simulink library "FlexBeamLib"  (R2019b)
settings: Solver=VariableStepAuto  StartTime=0.0  StopTime=10.0  RelTol=1e-3
undefined symbols (not defined in the file or in its folder): b, E, h, Izz, L, Mb, R, X, Y, Z
libraries: $bdroot x15, sm_lib x7
settings Model: Creator=tordaso  LastModifiedBy=tordaso

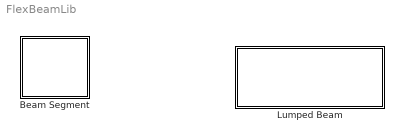
== system FlexBeamLib ==
  Beam Segment : Subsystem  mask{m=1, L=1, b=0.06, h=0.06, k=1000, c=10}
      mask prompts: m "Mass"; L "Length"; b "Width"; h "Height"; k "Joint Stiffness"; c "Joint Damping"
  Lumped Beam : Subsystem  mask{m=Mb(1), L=L(1), b=b(1), h=h(1), Izz=Izz(1), R=R, N=15, E=E}
      mask prompts: m "Mass"; L "Length"; b "Width"; h "Height"; R "Damping ratio"; N "Number of Elements"; E "E-Modulus"
      mask init:
      | % Get haandles of blocks and lines
      | blk = gcb;
      | blks = find_system(blk,...
      |     'LookUnderMasks','on',...
      |     'FollowLinks','on',...
      |     'FindAll', 'on'...
      | );
      | 
      | % Cleanup
      | for i = 2:length(blks)
      |     try
      |         type = get_param(blks(i), 'Type');
      |         name = get_param(blks(i), 'Name');
      |         
      |         if strcmp(type, 'line')
      |             delete_line(blks(i));
      |         end
      |         
      |         if strcmp(type, 'block')
      |             if strcmp(name, 'B')
      |                 hB = blks(i);
      |             elseif strcmp(name, 'F')
      |                 hF = blks(i);
      |             else
      |                 delete_block(blks(i));
      |             end
      |         end 
      |     end
      | end
      | 
      | % Beam segment paramters
      | mi = m/N;
      | Li = L/N;
      | bi = b;
      | hi = h;
      | ki = N*E*Izz/L;
      | ci = R*ki;
      | 
      | 
      | % Build N beam model
      | set_param([blk, '/B'], 'Position', flexlib.blockPos(0, 0, 30, 14));
      | for i = 1:N
      |     hBody = add_block('FlexBeamLib/Beam Segment',...
      |         [blk, '/body', num2str(i)],...
      |         'Position', flexlib.blockPos(70*i, 0, 40, 40)...
      |     );
      | 
      |     % Add lines
      |     if i > 1
      |         src = ['body', num2str(i-1), '/RConn1'];
      |         dst = ['body', num2str(i), '/LConn1'];
      |         
      |         add_line(blk, src, dst);
      |     end
      |     
      |     % Set parameters
      |     set_param(hBody, 'm', num2str(mi));
      |     set_param(hBody, 'L', num2str(Li));
      |     set_param(hBody, 'b', num2str(bi));
      |     set_param(hBody, 'h', num2str(hi));
      |     set_param(hBody, 'k', num2str(ki));
      |     set_param(hBody, 'c', num2str(ci));
      | 
      | end
      | 
      | % Move F
      | set_param([blk, '/F'], 'Position', flexlib.blockPos(70 + N*70, 0, 30, 14));
      | 
      | % Connect B and F
      | add_line(blk, 'B/RConn1', 'body1/LConn1');
      | add_line(blk, ['body', num2str(N), '/RConn1'], 'F/RConn1');

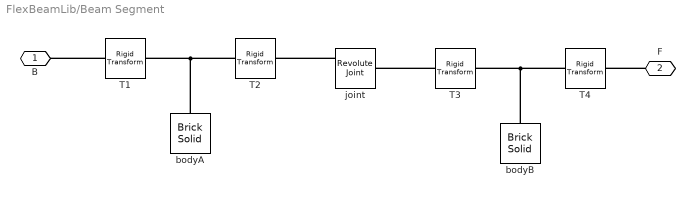
== system FlexBeamLib/Beam Segment ==
  T{1..4} (4 alike) : sm_lib/Frames and Transforms/Rigid Transform  TranslationMethod=Cartesian  TranslationStandardOffset=0  TranslationLengthUnit=m  TranslationStandardAxis=+Z  TranslationCartesianOffset=[L/4 0 0]  TranslationROffset=0  TranslationROffsetUnits=m  TranslationZOffset=0  TranslationZOffsetUnits=m  TranslationThetaOffset=0  TranslationThetaOffsetUnits=deg  RotationMethod=None  RotationAngleUnits=deg  RotationStandardAxis=+Z  RotationAngle=0.0  RotationArbitraryAxis=[0 0 1]  FollAlignAxisA=+X  BaseAlignAxisA=+Y  FollAlignAxisB=+Y  BaseAlignAxisB=+Z  RotationSequenceAxes=FollowerAxes  RotationSequence=XYX  RotationSequenceAngles=[0 0 0]  RotationSequenceAnglesUnits=deg  RotationMatrix=[1 0 0; 0 1 0; 0 0 1]
  bodyA : sm_lib/Body Elements/Brick Solid  GraphicAmbientColor=[0.15 0.15 0.15 1.0]  BasedOnType=Mass  BrickDimensions=[L/2 h b]  BrickDimensionUnits=m  CenterOfMass=[0 0 0]  CenterOfMassUnits=m  GraphicDiffuseColor=[0.0 0.0 0.0]  Density=1000  DensityUnits=kg/m^3  DoExposeReferenceFrame=on  GraphicEmissiveColor=[0.0 0.0 0.0 1.0]  ExportEntireGeometry=off  SerializedFrames=<Frames/>  MarkerShape=Sphere  MarkerSize=10  GraphicType=FromGeometry  InertiaType=CalculateFromGeometry  Mass=m  MassUnits=kg  MomentsOfInertia=[1 1 1]  MomentsOfInertiaUnits=kg*m^2  GraphicOpacity=1.0  ProductsOfInertia=[0 0 0]  ProductsOfInertiaUnits=kg*m^2  GraphicShininess=75  GraphicSpecularColor=[0.5 0.5 0.5 1.0]  GraphicVisPropType=SimpleVisualProperties
  bodyB : sm_lib/Body Elements/Brick Solid  GraphicAmbientColor=[0.15 0.15 0.15 1.0]  BasedOnType=Mass  BrickDimensions=[L/2 h b]  BrickDimensionUnits=m  CenterOfMass=[0 0 0]  CenterOfMassUnits=m  GraphicDiffuseColor=[1.0 1.0 0.0]  Density=1000  DensityUnits=kg/m^3  DoExposeReferenceFrame=on  GraphicEmissiveColor=[0.0 0.0 0.0 1.0]  ExportEntireGeometry=off  SerializedFrames=<Frames/>  MarkerShape=Sphere  MarkerSize=10  GraphicType=FromGeometry  InertiaType=CalculateFromGeometry  Mass=m  MassUnits=kg  MomentsOfInertia=[1 1 1]  MomentsOfInertiaUnits=kg*m^2  GraphicOpacity=1.0  ProductsOfInertia=[0 0 0]  ProductsOfInertiaUnits=kg*m^2  GraphicShininess=75  GraphicSpecularColor=[0.5 0.5 0.5 1.0]  GraphicVisPropType=SimpleVisualProperties
  joint : sm_lib/Joints/Revolute Joint  JointMode=Normal  SenseConstraintForce=off  SenseConstraintForceX=off  SenseConstraintForceY=off  SenseConstraintForceZ=off  SenseConstraintTorque=off  SenseConstraintTorqueX=off  SenseConstraintTorqueY=off  SenseConstraintTorqueZ=off  SenseTotalForce=off  SenseTotalForceX=off  SenseTotalForceY=off  SenseTotalForceZ=off  SenseTotalTorque=off  SenseTotalTorqueX=off  SenseTotalTorqueY=off  SenseTotalTorqueZ=off  CompositeWrenchDir=FollowerOnBase  CompositeWrenchFrame=BaseFrame  EquilibriumPosition=0  EquilibriumPositionUnits=deg  SpringStiffness=k  SpringStiffnessUnits=N*m/rad  DampingCoefficient=c  DampingCoefficientUnits=N*m/(rad/s)  TorqueActuationMode=InputTorque  MotionActuationMode=ComputedMotion  SensePosition=off  SenseVelocity=off  SenseAcceleration=off  SenseTorqueForce=off  SenseLowerLimitTorqueForce=off  SenseUpperLimitTorqueForce=off  LowerLimitSpecify=off  LowerLimitBound=-90  LowerLimitBoundUnits=deg  LowerLimitStiffness=1e4  LowerLimitStiffnessUnits=N*m/deg  LowerLimitDamping=10  LowerLimitDampingUnits=N*m/(deg/s)  LowerLimitTransitionRegionWidth=0.1  LowerLimitTransitionRegionWidthUnits=deg  UpperLimitSpecify=off  UpperLimitBound=90  UpperLimitBoundUnits=deg  UpperLimitStiffness=1e4  UpperLimitStiffnessUnits=N*m/deg  UpperLimitDamping=10  UpperLimitDampingUnits=N*m/(deg/s)  UpperLimitTransitionRegionWidth=0.1  UpperLimitTransitionRegionWidthUnits=deg  PositionTargetSpecify=off  PositionTargetPriority=High  PositionTargetValue=0  PositionTargetValueUnits=deg  VelocityTargetSpecify=off  VelocityTargetPriority=High  VelocityTargetValue=0  VelocityTargetValueUnits=deg/s
  B : PMIOPort  Side=Left
  F : PMIOPort  Port=2  Side=Right
  connections:
  T1/LConn1 -- B/RConn1
  bodyA/RConn1 -- T2/LConn1 -- T1/RConn1
  joint/LConn1 -- T2/RConn1
  bodyB/RConn1 -- T4/LConn1 -- T3/RConn1
  F/RConn1 -- T4/RConn1
  T3/LConn1 -- joint/RConn1

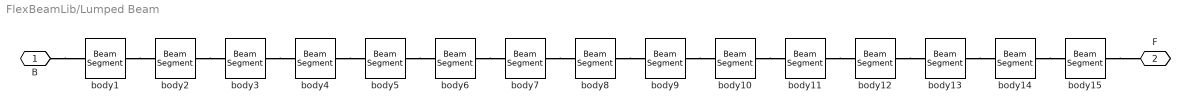
== system FlexBeamLib/Lumped Beam ==
  body{1..15} (15 alike) : $bdroot/Beam Segment  m=0.23328  L=0.1  b=0.075  h=0.075  k=523454.4  c=26172.72
  B : PMIOPort  Side=Left
  F : PMIOPort  Port=2  Side=Right
  connections:
  body15/RConn1 -- F/RConn1
  B/RConn1 -- body1/LConn1
  body14/RConn1 -- body15/LConn1
  body13/RConn1 -- body14/LConn1
  body12/RConn1 -- body13/LConn1
  body11/RConn1 -- body12/LConn1
  body10/RConn1 -- body11/LConn1
  body9/RConn1 -- body10/LConn1
  body8/RConn1 -- body9/LConn1
  body7/RConn1 -- body8/LConn1
  body6/RConn1 -- body7/LConn1
  body5/RConn1 -- body6/LConn1
  body4/RConn1 -- body5/LConn1
  body3/RConn1 -- body4/LConn1
  body2/RConn1 -- body3/LConn1
  body1/RConn1 -- body2/LConn1
